simulink model "Project_4_Simulink"  (R2023b)
settings: Solver=ode45  StartTime=0.0  StopTime=3600  MaxStep=5.0  RelTol=1e-3
undefined symbols (not defined in the file or in its folder): batData, carData, motorData, track_radius
libraries: slpidlib x1
settings Model: NumberOfSteps=100  Creator=Matt Cain  LastModifiedBy=xavie

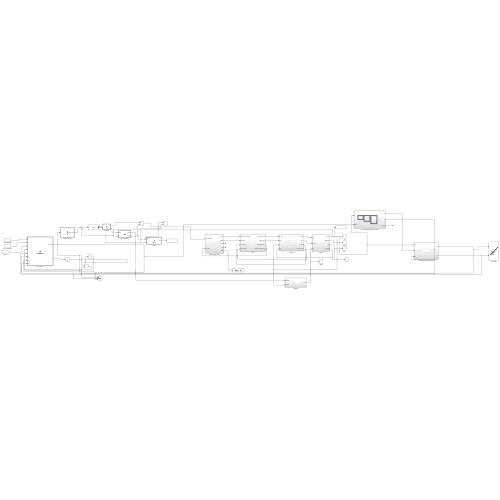
[thumbnail: Simulink's stored preview of the top-level diagram]
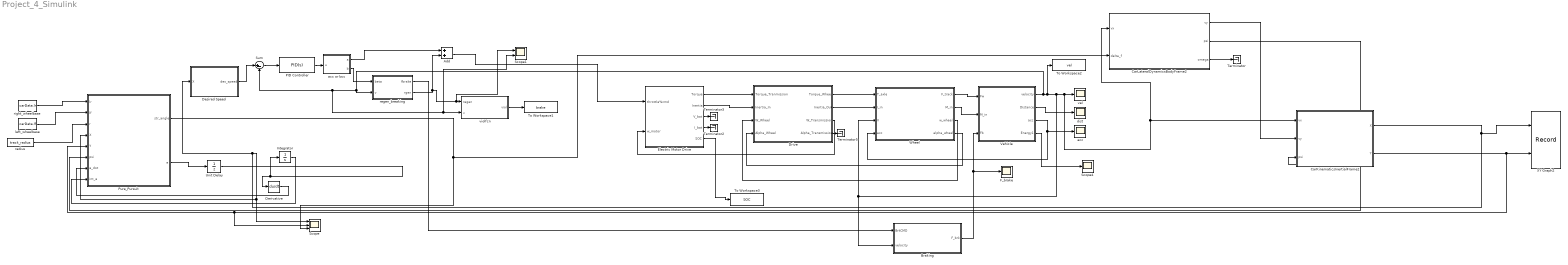
== system Project_4_Simulink ==
  Add : Sum
  Braking : Subsystem
  CarKinematicsInertialFrame2 : Subsystem
  CarLateralDynamicsBodyFrame2 : Subsystem
  Derivative : Derivative
  Desired Speed : MATLAB Function  TreatAsAtomicUnit=on
  Drive : Subsystem
  Electric Motor Drive : Subsystem
  F_brake : Scope
  Integrator : Integrator
  PID Controller : slpidlib/PID Controller  Controller=PID  Form=Parallel  TimeDomain=Continuous-time  UseExternalTs=off  SampleTime=-1  IntegratorMethod=Forward Euler  FilterMethod=Forward Euler  ControllerParametersSource=internal  P=0.1  I=0  UseKiTs=off  D=0  N=100  UseFilter=on  TunerSelectOption=Transfer Function Based (PID Tuner App)  InitialConditionSource=internal  InitialConditionForIntegrator=0  InitialConditionForFilter=0  DifferentiatorICPrevScaledInput=0  ExternalReset=none  TrackingMode=off  Kt=1  LimitOutput=on  SatLimitsSource=internal  UpperSaturationLimit=1  LowerSaturationLimit=-1  LinearizeAsGain=off  AntiWindupMode=none  Kb=1  LimitIntegrator=off  UpperIntegratorSaturationLimit=inf  LowerIntegratorSaturationLimit=-inf  POutMin=[]  POutMax=[]  IOutMin=[]  IOutMax=[]  DOutMin=[]  DOutMax=[]  NOutMin=[]  NOutMax=[]  SumOutMin=[]  SumOutMax=[]  SaturationOutMin=[]  SaturationOutMax=[]  PParamMin=[]  PParamMax=[]  IParamMin=[]  IParamMax=[]  DParamMin=[]  DParamMax=[]  NParamMin=[]  NParamMax=[]  KbParamMin=[]  KbParamMax=[]  KtParamMin=[]  KtParamMax=[]  KbOutMin=[]  KbOutMax=[]  KtOutMin=[]  KtOutMax=[]  IntegratorOutMin=[]  IntegratorOutMax=[]  FilterOutMin=[]  FilterOutMax=[]  SumI1OutMin=[]  SumI1OutMax=[]  SumI2OutMin=[]  SumI2OutMax=[]  SumI3OutMin=[]  SumI3OutMax=[]  SumI4OutMin=[]  SumI4OutMax=[]  SumDOutMin=[]  SumDOutMax=[]  DifferentiatorOutMin=[]  DifferentiatorOutMax=[]  FilterDiffOutCoefMin=[]  FilterDiffOutCoefMax=[]  ReciprocalOutMin=[]  ReciprocalOutMax=[]  SumDenOutMin=[]  SumDenOutMax=[]  SumNumOutMin=[]  SumNumOutMax=[]  DivideOutMin=[]  DivideOutMax=[]  UdiffTsProdOutMin=[]  UdiffTsProdOutMax=[]  NTsProdOutMin=[]  NTsProdOutMax=[]  UintegralTsProdOutMin=[]  UintegralTsProdOutMax=[]  UngainTsProdOutMin=[]  UngainTsProdOutMax=[]  ClampingZeroOutDataTypeStr=Inherit: Inherit via back propagation  ClampingZeroOutMin=[]  ClampingZeroOutMax=[]  FilterDenConstantOutDataTypeStr=Inherit: Inherit via back propagation  FilterDenConstantOutMin=[]  FilterDenConstantOutMax=[]  PCopyOutDataTypeStr=Inherit: Inherit via back propagation  PCopyOutMin=[]  PCopyOutMax=[]  NCopyOutDataTypeStr=Inherit: Inherit via back propagation  NCopyOutMin=[]  NCopyOutMax=[]  IntegratorContinuousStateAttributes=''  IntegratorStateMustResolveToSignalObject=off  IntegratorRTWStateStorageClass=Auto  FilterContinuousStateAttributes=''  FilterStateMustResolveToSignalObject=off  FilterRTWStateStorageClass=Auto  ParallelPVariant=InternalParameters  IdealPVariant=Disabled  IVariant=InternalParameters  DVariant=InternalParameters  IntegratorVariant=Continuous  SatVariant=Enabled  AWVariant=Passthrough  PCopyVariant=Disabled  TRVariant=Disabled  FdbkBlocksVariant=Forward  IdealPFdbkVariant=Disabled  SatFdbkVariant=Disabled  DerivativeFilterVariant=ContFilter  NVariant=InternalParameters  NCopyVariant=Disabled  FilterICVariant=InternalICsFilter  IntegratorICVariant=InternalICs  ExternalResetVariant=Disabled  TRSumVariant=Passthrough  SumFdbkVariant=Disabled  SumVariant=Sum_PID  TsampFilterVariant=InternalTs  TsampNgainVariant=Passthrough  TsampIntegralVariant=Disabled_SignalSpec  ExternalSaturationOutDataTypeStr=Inherit: Same as second input
  Pure_Pursuit : MATLAB Function  TreatAsAtomicUnit=on
  Scope : Scope  NumInputPorts=3
  Scope1 : Scope  NumInputPorts=2
  Scope4 : Scope
  Sum : Sum  Inputs=|+-
  Terminator{,2..3,5} (4 alike) : Terminator
  To Workspace1 : ToWorkspace  VariableName=brake  SaveFormat=Timeseries  SampleTime=-1
  To Workspace2 : ToWorkspace  VariableName=vel  SaveFormat=Timeseries  SampleTime=-1
  To Workspace3 : ToWorkspace  VariableName=SOC  SaveFormat=Timeseries  SampleTime=-1
  Unit Delay : UnitDelay  SampleTime=-1  HasFrameUpgradeWarning=on
  Vehicle : Subsystem
  "Wheel " : Subsystem
  XY Graph2 : Record  FileSettingsInternal="{\"entries\":[{\"content\":{\"excelSettings\":{\"content\":{},\"type\":\"Streamout.ExcelSettings\"}},\"type\":\"Streamout.FileSettingStorage\",\"uuid\":\"\"}],\"packageUris\":[\"http:\\/\\/schema.mathworks.com\\/mf0\\/streamout_blocks\\/R2020a\"],\"version\":\"1.0\"}"  Layout=[1 1]  SignalsInternal="{\"entries\":[{\"content\":{\"signals\":[{\"content\":{\"blockPath\":[],\"dimensions\":[1],\"domain\":\"\",\"lineColor\":\"#edb120\",\"port\":1,\"sid\":[\"\"],\"signalID\":23658,\"signalName\":\"CarKinematicsInertialFrame2:1\"},\"type\":\"RecordBlkView.Signal\",\"uuid\":\"\"},{\"content\":{\"blockPath\":[],\"dimensions\":[1],\"domain\":\"\",\"lineColor\":\"#7e2f8e\",\"port\":2,\"sid\":[\"\"],\"signalID\":23662,\"signalName\":\"CarKinematicsInertialFrame2:2\"},\"type\":\"RecordBlkView.Signal\",\"uuid\":\"\"}]},\"type\":\"RecordBlkView.InputSignals\",\"uuid\":\"\"}],\"packageUris\":[\"http:\\/\\/schema.mathworks.com\\/mf0\\/streamout_blocks\\/R2020a\"],\"version\":\"1.0\"}"  VisualizationBindings="{\"xyplotplugin\":{\"info\":[{\"series\":[{\"bindingParametersList\":[{\"parameter\":\"X-Axis\",\"signalID\":23062,\"signalName\":\"CarKinematicsInertialFrame2:1\"},{\"parameter\":\"Y-Axis\",\"signalID\":23066,\"signalName\":\"CarKinematicsInertialFrame2:2\"}],\"seriesID\":49385}],\"subplotID\":1}]}}"  CompatibilityTag=XY  st=-1
  acc : Scope
  acc or bcc : MATLAB Function  TreatAsAtomicUnit=on
  dist : Scope
  left_wheelbase : Constant  Value=carData.lf
  radius : Constant  Value=track_radius
  regen_breaking : MATLAB Function  TreatAsAtomicUnit=on
  right_wheelbase : Constant  Value=carData.lr
  vel : Scope
  violfcn : MATLAB Function  TreatAsAtomicUnit=on
  wires:
  acc or bcc/2(b) -> regen_breaking/1(beta)
  CarKinematicsInertialFrame2/1(X) -> Desired Speed/1(X), Scope/1, Pure_Pursuit/4(X), XY Graph2/1
  regen_breaking/2(rgen) -> Add/2, Scope1/1, violfcn/1(regen)
  Pure_Pursuit/1(str_angle) -> CarLateralDynamicsBodyFrame2/2(delta_f), Scope/3
  Sum/1 -> PID Controller/1
  violfcn/1(viol) -> To Workspace1/1
  Integrator/1 -> Pure_Pursuit/8(int_e)
  right_wheelbase/1 -> Pure_Pursuit/1(lr)
  CarLateralDynamicsBodyFrame2/2(psi) -> Pure_Pursuit/6(psi), CarKinematicsInertialFrame2/3(psi)
  CarKinematicsInertialFrame2/2(Y) -> XY Graph2/2, Pure_Pursuit/5(Y), Scope/2
  Pure_Pursuit/2(e) -> Unit Delay/1
  left_wheelbase/1 -> Pure_Pursuit/2(lf)
  Unit Delay/1 -> Derivative/1, Integrator/1
  acc or bcc/1(a) -> Add/1
  Derivative/1 -> Pure_Pursuit/7(e_dot)
  radius/1 -> Pure_Pursuit/3(r)
  Vehicle/1("velocity ") -> Sum/2, Scope1/2, violfcn/2(v), regen_breaking/2(v), To Workspace2/1, CarLateralDynamicsBodyFrame2/1(vx), CarKinematicsInertialFrame2/1(vx), vel/1, Braking/2("velocity "), "Wheel "/3(V)
  PID Controller/1 -> acc or bcc/1(u)
  Desired Speed/1(des_speed) -> Sum/1
  "Wheel "/3(w_wheel) -> Drive/3(W_Wheel)
  regen_breaking/1(fbrake) -> Braking/1("BrkCMD ")
  "Wheel "/4(alpha_wheel) -> Drive/4(Alpha_Wheel)
  Drive/4(Alpha_Transmission) -> Terminator5/1
  "Wheel "/2(M_in) -> Vehicle/2("M_in ")
  Electric Motor Drive/5(SOC) -> To Workspace3/1
  Vehicle/2("Distance ") -> dist/1
  Electric Motor Drive/2(Inertia) -> Drive/2(Inertia_In)
  Electric Motor Drive/4(I_bat) -> Terminator2/1
  Electric Motor Drive/1(Torque) -> Drive/1(Torque_Tranmission)
  Vehicle/3(acc) -> acc/1, "Wheel "/4(acc)
  "Wheel "/1(F_track) -> Vehicle/1("Fw ")
  Drive/3(W_Transmission) -> Electric Motor Drive/2(w_motor)
  Electric Motor Drive/3(V_bat) -> Terminator3/1
  Braking/1("F_brk ") -> Vehicle/3("Fb "), F_brake/1
  Drive/2(Inertia_Out) -> "Wheel "/2(I_in)
  Drive/1(Torque_Wheel) -> "Wheel "/1(T_axle)
  CarLateralDynamicsBodyFrame2/1(vy) -> CarKinematicsInertialFrame2/2(vy)
  Add/1 -> Electric Motor Drive/1(throttle%cmd)
  CarLateralDynamicsBodyFrame2/3(omega) -> Terminator/1
  Vehicle/4(Energy1) -> Scope4/1

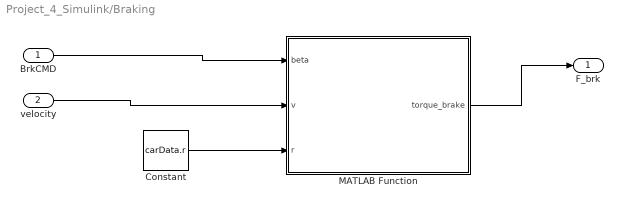
== system Project_4_Simulink/Braking ==
  "BrkCMD " : Inport
  "velocity " : Inport  Port=2
  Constant : Constant  Value=carData.r
  MATLAB Function : MATLAB Function  TreatAsAtomicUnit=on
  "F_brk " : Outport  VectorParamsAs1DForOutWhenUnconnected=off
  wires:
  "BrkCMD "/1 -> MATLAB Function/1(beta)
  MATLAB Function/1(torque_brake) -> "F_brk "/1
  "velocity "/1 -> MATLAB Function/2(v)
  Constant/1 -> MATLAB Function/3(r)

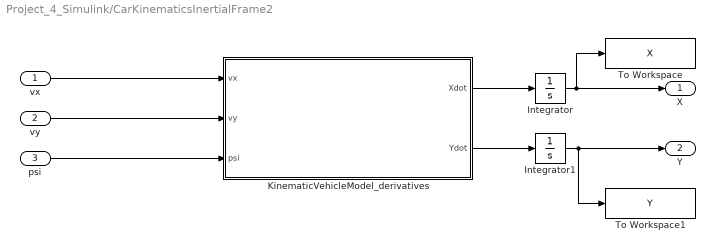
== system Project_4_Simulink/CarKinematicsInertialFrame2 ==
  vx : Inport
  vy : Inport  Port=2
  psi : Inport  Port=3
  Integrator : Integrator  InitialCondition=carData.init.X0
  Integrator1 : Integrator  InitialCondition=carData.init.Y0
  KinematicVehicleModel_derivatives : MATLAB Function  TreatAsAtomicUnit=on  mask{obj=carData}
      mask prompts: obj "obj structure"
  To Workspace : ToWorkspace  VariableName=X  SaveFormat=Structure With Time  SampleTime=-1
  To Workspace1 : ToWorkspace  VariableName=Y  SaveFormat=Structure With Time  SampleTime=-1
  X : Outport
  Y : Outport  Port=2
  wires:
  KinematicVehicleModel_derivatives/1(Xdot) -> Integrator/1
  KinematicVehicleModel_derivatives/2(Ydot) -> Integrator1/1
  Integrator/1 -> To Workspace/1, X/1
  Integrator1/1 -> To Workspace1/1, Y/1
  vx/1 -> KinematicVehicleModel_derivatives/1(vx)
  vy/1 -> KinematicVehicleModel_derivatives/2(vy)
  psi/1 -> KinematicVehicleModel_derivatives/3(psi)

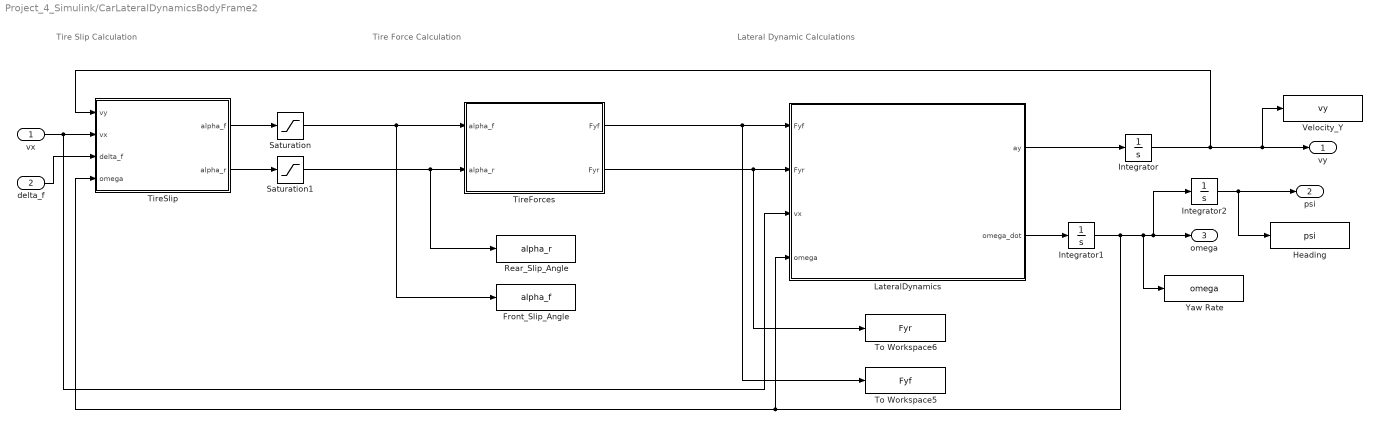
== system Project_4_Simulink/CarLateralDynamicsBodyFrame2 ==
  note: Tire Slip Calculation
  note: Tire Force Calculation
  note: Lateral Dynamic Calculations
  vx : Inport
  delta_f : Inport  Port=2
  Front_Slip_Angle : ToWorkspace  VariableName=alpha_f  SaveFormat=Timeseries  SampleTime=-1
  Heading : ToWorkspace  VariableName=psi  SaveFormat=Timeseries  SampleTime=-1
  Integrator : Integrator  InitialCondition=carData.init.vy0
  Integrator1 : Integrator  InitialCondition=carData.init.omega0
  Integrator2 : Integrator  InitialCondition=carData.init.psi0
  LateralDynamics : MATLAB Function  TreatAsAtomicUnit=on  mask{obj=carData}
      mask prompts: obj "obj structure"
  Rear_Slip_Angle : ToWorkspace  VariableName=alpha_r  SaveFormat=Timeseries  SampleTime=-1
  Saturation : Saturate  UpperLimit=carData.maxAlpha  LowerLimit=-carData.maxAlpha
  Saturation1 : Saturate  UpperLimit=carData.maxAlpha  LowerLimit=-carData.maxAlpha
  TireForces : MATLAB Function  TreatAsAtomicUnit=on  mask{obj=carData}
      mask prompts: obj "obj structure"
  TireSlip : MATLAB Function  TreatAsAtomicUnit=on  mask{obj=carData}
      mask prompts: obj "obj structure"
  To Workspace5 : ToWorkspace  VariableName=Fyf  SaveFormat=Timeseries  SampleTime=-1
  To Workspace6 : ToWorkspace  VariableName=Fyr  SaveFormat=Timeseries  SampleTime=-1
  Velocity_Y : ToWorkspace  VariableName=vy  SaveFormat=Timeseries  SampleTime=-1
  Yaw Rate : ToWorkspace  VariableName=omega  SaveFormat=Timeseries  SampleTime=-1
  vy : Outport
  psi : Outport  Port=2
  omega : Outport  Port=3
  wires:
  LateralDynamics/1(ay) -> Integrator/1
  Integrator/1 -> vy/1, Velocity_Y/1, TireSlip/1(vy)
  LateralDynamics/2(omega_dot) -> Integrator1/1
  Integrator1/1 -> Integrator2/1, omega/1, Yaw Rate/1, LateralDynamics/4(omega), TireSlip/4(omega)
  TireSlip/1(alpha_f) -> Saturation/1
  TireSlip/2(alpha_r) -> Saturation1/1
  TireForces/1(Fyf) -> LateralDynamics/1(Fyf), To Workspace5/1
  TireForces/2(Fyr) -> LateralDynamics/2(Fyr), To Workspace6/1
  Saturation/1 -> TireForces/1(alpha_f), Front_Slip_Angle/1
  Saturation1/1 -> TireForces/2(alpha_r), Rear_Slip_Angle/1
  vx/1 -> TireSlip/2(vx), LateralDynamics/3(vx)
  delta_f/1 -> TireSlip/3(delta_f)
  Integrator2/1 -> Heading/1, psi/1

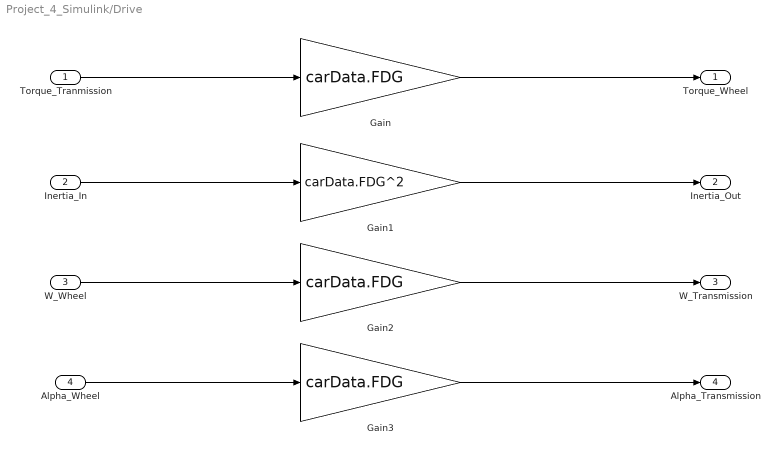
== system Project_4_Simulink/Drive ==
  Torque_Tranmission : Inport
  Inertia_In : Inport  Port=2
  W_Wheel : Inport  Port=3
  Alpha_Wheel : Inport  Port=4
  Gain : Gain  Gain=carData.FDG
  Gain1 : Gain  Gain=carData.FDG^2
  Gain2 : Gain  Gain=carData.FDG
  Gain3 : Gain  Gain=carData.FDG
  Torque_Wheel : Outport
  Inertia_Out : Outport  Port=2
  W_Transmission : Outport  Port=3
  Alpha_Transmission : Outport  Port=4
  wires:
  Torque_Tranmission/1 -> Gain/1
  Inertia_In/1 -> Gain1/1
  W_Wheel/1 -> Gain2/1
  Alpha_Wheel/1 -> Gain3/1
  Gain/1 -> Torque_Wheel/1
  Gain1/1 -> Inertia_Out/1
  Gain2/1 -> W_Transmission/1
  Gain3/1 -> Alpha_Transmission/1

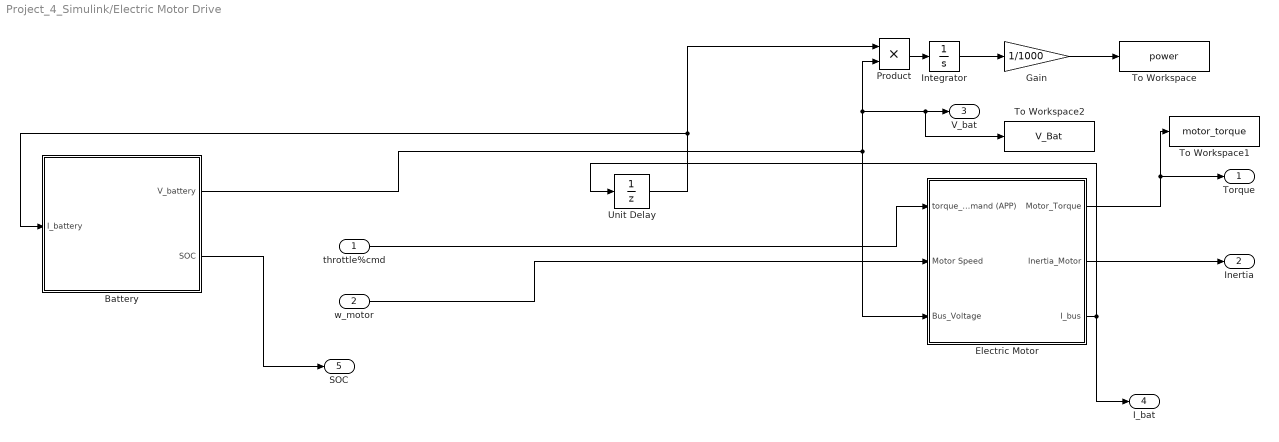
== system Project_4_Simulink/Electric Motor Drive ==
  throttle%cmd : Inport
  w_motor : Inport  Port=2
  Battery : Subsystem
  Electric Motor : Subsystem
  Gain : Gain  Gain=1/1000
  Integrator : Integrator
  Product : Product
  To Workspace : ToWorkspace  VariableName=power  SaveFormat=Timeseries  SampleTime=-1
  To Workspace1 : ToWorkspace  VariableName=motor_torque  SaveFormat=Timeseries  SampleTime=-1
  To Workspace2 : ToWorkspace  VariableName=V_Bat  SaveFormat=Timeseries  SampleTime=-1
  Unit Delay : UnitDelay  SampleTime=-1  HasFrameUpgradeWarning=on
  Torque : Outport
  Inertia : Outport  Port=2
  V_bat : Outport  Port=3
  I_bat : Outport  Port=4
  SOC : Outport  Port=5
  wires:
  throttle%cmd/1 -> Electric Motor/1(torque_Command (APP))
  w_motor/1 -> Electric Motor/2(Motor Speed)
  Electric Motor/3(I_bus) -> Unit Delay/1, I_bat/1
  Battery/1(V_battery) -> To Workspace2/1, V_bat/1, Product/2, Electric Motor/3(Bus_Voltage)
  Battery/2(SOC) -> SOC/1
  Electric Motor/2(Inertia_Motor) -> Inertia/1
  Electric Motor/1(Motor_Torque) -> To Workspace1/1, Torque/1
  Unit Delay/1 -> Battery/1(I_battery), Product/1
  Product/1 -> Integrator/1
  Integrator/1 -> Gain/1
  Gain/1 -> To Workspace/1

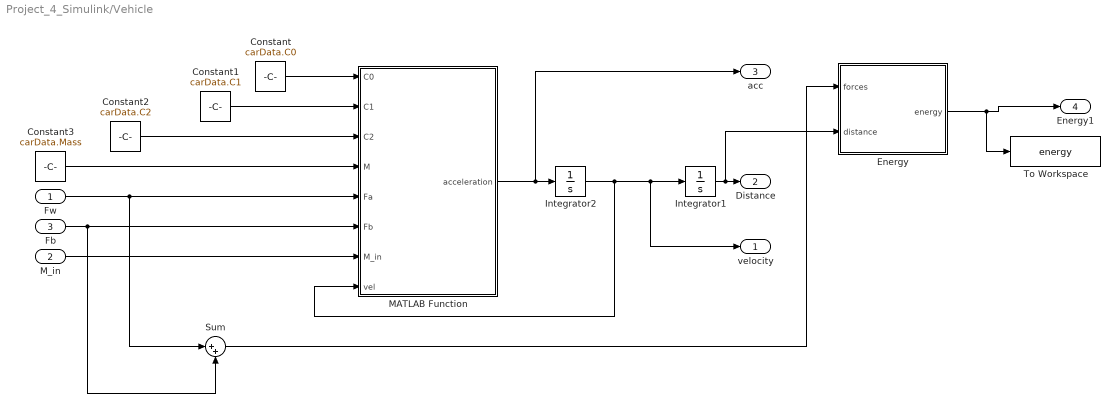
== system Project_4_Simulink/Vehicle ==
  "Fw " : Inport
  "M_in " : Inport  Port=2
  "Fb " : Inport  Port=3
  Constant : Constant  Value=carData.C0
  Constant1 : Constant  Value=carData.C1
  Constant2 : Constant  Value=carData.C2
  Constant3 : Constant  Value=carData.Mass
  Energy : MATLAB Function  TreatAsAtomicUnit=on
  Integrator1 : Integrator
  Integrator2 : Integrator  LimitOutput=on  LowerSaturationLimit=0
  MATLAB Function : MATLAB Function  TreatAsAtomicUnit=on
  Sum : Sum  Inputs=|++
  To Workspace : ToWorkspace  VariableName=energy  SaveFormat=Timeseries  SampleTime=-1
  "velocity " : Outport  VectorParamsAs1DForOutWhenUnconnected=off
  "Distance " : Outport  Port=2  VectorParamsAs1DForOutWhenUnconnected=off
  acc : Outport  Port=3
  Energy1 : Outport  Port=4
  wires:
  Constant1/1 -> MATLAB Function/2(C1)
  Constant/1 -> MATLAB Function/1(C0)
  Constant2/1 -> MATLAB Function/3(C2)
  Constant3/1 -> MATLAB Function/4(M)
  "Fw "/1 -> Sum/1, MATLAB Function/5(Fa)
  "Fb "/1 -> Sum/2, MATLAB Function/6(Fb)
  Integrator1/1 -> Energy/2(distance), "Distance "/1
  "M_in "/1 -> MATLAB Function/7(M_in)
  MATLAB Function/1(acceleration) -> acc/1, Integrator2/1
  Integrator2/1 -> MATLAB Function/8(vel), "velocity "/1, Integrator1/1
  Sum/1 -> Energy/1(forces)
  Energy/1(energy) -> To Workspace/1, Energy1/1

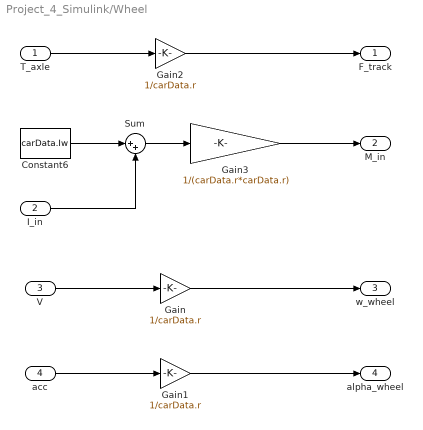
== system Project_4_Simulink/Wheel  ==
  T_axle : Inport
  I_in : Inport  Port=2
  V : Inport  Port=3
  acc : Inport  Port=4
  Constant6 : Constant  Value=carData.Iw
  Gain : Gain  Gain=1/carData.r
  Gain1 : Gain  Gain=1/carData.r
  Gain2 : Gain  Gain=1/carData.r
  Gain3 : Gain  Gain=1/(carData.r*carData.r)
  Sum : Sum  Inputs=|++
  F_track : Outport
  M_in : Outport  Port=2
  w_wheel : Outport  Port=3
  alpha_wheel : Outport  Port=4
  wires:
  Gain/1 -> w_wheel/1
  V/1 -> Gain/1
  acc/1 -> Gain1/1
  Gain1/1 -> alpha_wheel/1
  T_axle/1 -> Gain2/1
  Gain2/1 -> F_track/1
  Gain3/1 -> M_in/1
  Constant6/1 -> Sum/1
  I_in/1 -> Sum/2
  Sum/1 -> Gain3/1

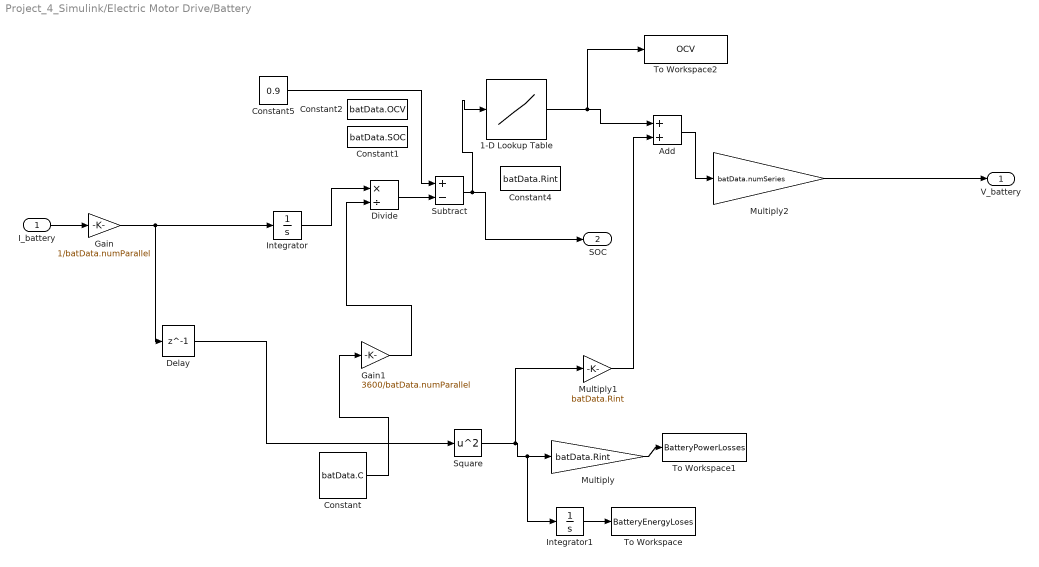
== system Project_4_Simulink/Electric Motor Drive/Battery ==
  I_battery : Inport
  1-D Lookup Table : Lookup_n-D  NumberOfTableDimensions=1  BreakpointsForDimension1=batData.SOC  Table=batData.OCV  InternalRulePriority=Speed  RndMeth=Simplest
  Add : Sum
  Constant : Constant  Value=batData.C
  Constant1 : Constant  Value=batData.SOC
  Constant2 : Constant  Value=batData.OCV
  Constant4 : Constant  Value=batData.Rint
  Constant5 : Constant  Value=0.9
  Delay : Delay  DelayLength=1
  Divide : Product  Inputs=*/
  Gain : Gain  Gain=1/batData.numParallel
  Gain1 : Gain  Gain=3600/batData.numParallel
  Integrator : Integrator
  Integrator1 : Integrator
  Multiply : Gain  Gain=batData.Rint
  Multiply1 : Gain  Gain=batData.Rint
  Multiply2 : Gain  Gain=batData.numSeries
  Square : Math  Operator=square
  Subtract : Sum  Inputs=+-
  To Workspace : ToWorkspace  VariableName=BatteryEnergyLoses  SaveFormat=Timeseries  SampleTime=-1
  To Workspace1 : ToWorkspace  VariableName=BatteryPowerLosses  SaveFormat=Timeseries  SampleTime=-1
  To Workspace2 : ToWorkspace  VariableName=OCV  SaveFormat=Timeseries  SampleTime=-1
  V_battery : Outport
  SOC : Outport  Port=2
  wires:
  I_battery/1 -> Gain/1
  Gain/1 -> Delay/1, Integrator/1
  Integrator/1 -> Divide/1
  Constant/1 -> Gain1/1
  Gain1/1 -> Divide/2
  Divide/1 -> Subtract/2
  Constant5/1 -> Subtract/1
  Subtract/1 -> 1-D Lookup Table/1, SOC/1
  Delay/1 -> Square/1
  Square/1 -> Multiply1/1, Integrator1/1, Multiply/1
  1-D Lookup Table/1 -> To Workspace2/1, Add/1
  Multiply1/1 -> Add/2
  Add/1 -> Multiply2/1
  Integrator1/1 -> To Workspace/1
  Multiply/1 -> To Workspace1/1
  Multiply2/1 -> V_battery/1

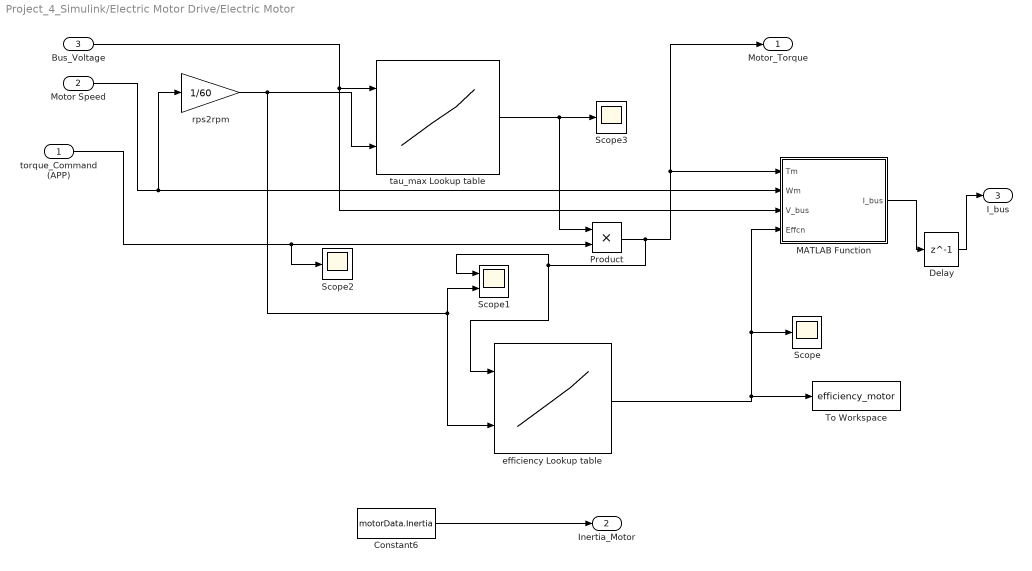
== system Project_4_Simulink/Electric Motor Drive/Electric Motor ==
  torque_Command (APP) : Inport
  Motor Speed : Inport  Port=2
  Bus_Voltage : Inport  Port=3
  Constant6 : Constant  Value=motorData.Inertia
  Delay : Delay  DelayLength=1
  MATLAB Function : MATLAB Function  TreatAsAtomicUnit=on
  Product : Product
  Scope : Scope
  Scope1 : Scope  NumInputPorts=2
  Scope2 : Scope
  Scope3 : Scope
  To Workspace : ToWorkspace  VariableName=efficiency_motor  SaveFormat=Timeseries  SampleTime=-1
  efficiency Lookup table : Lookup_n-D  BreakpointsForDimension1=motorData.eta_torque  BreakpointsForDimension2=motorData.eta_speed  BeginIndexSearchUsingPreviousIndexResult=on  Table=motorData.eta_val  InternalRulePriority=Speed  RndMeth=Simplest
      settings: InputPortMap=u0,u1
  rps2rpm : Gain  Gain=1/60
  tau_max Lookup table : Lookup_n-D  BreakpointsForDimension1=motorData.vbus  BreakpointsForDimension2=motorData.rpm  Table=motorData.maxtorque  InternalRulePriority=Speed  RndMeth=Simplest
      settings: InputPortMap=u0,u1
  Motor_Torque : Outport
  Inertia_Motor : Outport  Port=2
  I_bus : Outport  Port=3
  wires:
  Bus_Voltage/1 -> tau_max Lookup table/1, MATLAB Function/3(V_bus)
  torque_Command (APP)/1 -> Scope2/1, Product/2
  tau_max Lookup table/1 -> Product/1, Scope3/1
  Product/1 -> efficiency Lookup table/1, Scope1/1, MATLAB Function/1(Tm), Motor_Torque/1
  efficiency Lookup table/1 -> MATLAB Function/4(Effcn), Scope/1, To Workspace/1
  MATLAB Function/1(I_bus) -> Delay/1
  Constant6/1 -> Inertia_Motor/1
  Motor Speed/1 -> MATLAB Function/2(Wm), rps2rpm/1
  rps2rpm/1 -> Scope1/2, efficiency Lookup table/2, tau_max Lookup table/2
  Delay/1 -> I_bus/1

== matlab function Project_4_Simulink/CarLateralDynamicsBodyFrame2/LateralDynamics ==
  data: Fyf input; Fyr input size=1; vx input; omega input; ay output; obj parameter; omega_dot output
function [ay, omega_dot] = fcn(Fyf, Fyr, vx, omega, obj)

Fy = Fyf + Fyr;
ay = Fy / obj.Mass - omega * vx;
        
M  = Fyf * obj.lf - Fyr * obj.lr;        
omega_dot = M / obj.Inertia;        

end

== matlab function Project_4_Simulink/CarLateralDynamicsBodyFrame2/TireForces ==
  data: alpha_f input; alpha_r input; Fyf output; obj parameter; Fyr output
function [Fyf, Fyr] = fcn(alpha_f, alpha_r, obj)

Fyf = min(obj.Fyfmax,obj.Calpha_f * alpha_f);
Fyr = min(obj.Fyrmax, obj.Calpha_r * alpha_r);
end

== matlab function Project_4_Simulink/CarLateralDynamicsBodyFrame2/TireSlip ==
  data: vy input size=1; vx input; delta_f input size=1; omega input; alpha_f output; obj parameter; alpha_r output
function [alpha_f, alpha_r] = fcn(vy,  vx, delta_f, omega, obj)


if abs(vx)> obj.vx_threshold1
      alpha_f = delta_f - (vy + omega * obj.lf) / vx;
      alpha_r = - (vy - omega * obj.lr) / vx;
else
      alpha_f = 0;
      alpha_r = 0;
end



end

== matlab function Project_4_Simulink/CarKinematicsInertialFrame2/KinematicVehicleModel_derivatives ==
  data: vx input; vy input; psi input size=1; Xdot output; Ydot output
function [Xdot, Ydot] = fcn(vx, vy, psi)
    temp = TF(psi) * [vx;vy]; 
    Xdot = temp(1);
    Ydot = temp(2);
  
end

function y = TF(psi)
    y = [cos(psi), -sin(psi); sin(psi), cos(psi)];
end

== matlab function Project_4_Simulink/acc or bcc ==
  data: u input; a output; b output
% Checks if there is a difference between actual speed and desired speed

% u is calculated using the sum function in the simulink model

function [a,b] = fcn(u)

if u>0 % If the difference is greater than zero, then we need to speed up since actual speed is less than desired speed
    acc=u; % We send how much we need to speed up to the throttle command
    brk=0; % Do nothing for the break command
elseif u<0 % If the difference is less than zero, then we need to slow down since the actual speed is less than the desired speed
    acc=0; % Do nothing for throttle command
    brk=-u; % We send how much we need to break to the break command
else % If the desired and actual speed is the same
    acc=0; % Do nothing for throttle command
    brk=0; % Do nothing for the break command
end
a= acc; % storing how much acceleration required to a
b= brk; % storing how much break acceleration required to b

== matlab function Project_4_Simulink/Pure_Pursuit ==
  data: lr input; lf input; r input; X input; str_angle output; Y input; psi input; e_dot input; int_e input; e output
function [str_angle, e] = SimplestDriver(lr, lf, r, X, Y, psi, e_dot, int_e)
lookout = 10;
kp = .0017;
kd = 0;
ki = 0;
if X >= 900
    theta = atan(200-Y/X-900);
    psi_desired = psi+theta;
    e = psi - psi_desired;
    PID = kp*e + kd*e_dot + ki*int_e;
    str_angle = PID + (lr+lf)/r;
elseif X < 0
    theta = atan(200-Y/X - 900);
    psi_desired = psi+theta;
    e = psi - psi_desired;
    PID = kp*e + kd*e_dot + ki*int_e;
    str_angle = PID + (lr+lf)/r;
else
    str_angle = 0;
    psi_desired = 0;
    e = psi-psi_desired;
    kp = 0.00050;
    kd = 0.0007/1000000;
    ki = 0.00000000011/100000000;
    if Y < 200
        lookout= 45;
        vertical = -Y;
        psi_desired = atan(vertical/lookout);
        e = psi_desired;
        PID = kp*e + kd*e_dot + ki*int_e;
        str_angle = PID;
    end
    if Y > 200
        lookout= -45;
        vertical = 400-Y;
        psi_desired = atan(vertical/lookout);
        e = psi_desired;
        PID = kp*e + kd*e_dot + ki*int_e;
        str_angle = PID;
    end
end

== matlab function Project_4_Simulink/Desired Speed ==
  data: X input; des_speed output
function des_speed = fcn(X)
if X > 0  && X <15 || X < 900 && X > 885
    des_speed = 70;
elseif X <= 885 && X >= 15
    des_speed = 80;
else
    des_speed = 10.5;
end

== matlab function Project_4_Simulink/violfcn ==
  data: regen input; viol output; v input

function viol = violfcn(regen, v)
    speed = v ;%* (3600/1600);
    if speed < 5
        regen_vio = 0;
        if abs(regen -regen_vio ) < 1E-6
            viol = 0;
        else
            viol = 1;
        end

    elseif speed == 25
        regen_vio = 0.95;
        if abs(regen - regen_vio ) < 1E-6
            viol = 0;
        else
            viol = 1;
        end

    elseif speed > 25
        regen_vio = 0.95;
        if abs(regen -regen_vio ) < 1E-6
            viol = 0;
        else
            viol = 1;
        end
    else
        regen_vio = ((0.95/20)*speed) - 0.2375;
        if abs(regen -regen_vio ) < 1E-6
            viol = 0;
        else
            viol = 1;
        end
    end

== matlab function Project_4_Simulink/regen_breaking ==
  data: fbrake output; beta input; v input; rgen output
% function [fbrake, rgen] = fcn(beta, v)
function [fbrake, rgen]= fcn(beta, v)
%speed = v * (3600/1600);
%v = speed;
if v <= 5
    rgen = 0;
    fbrake = beta;
elseif v > 5
    rgen = .0475 * ((v-5)*beta);
    fbrake = ( 1-0.0475)*((v-5)*beta);
else
    rgen = 0.05*beta;
    fbrake = 0.95*beta;
end

== matlab function Project_4_Simulink/Braking/MATLAB Function ==
  data: beta input; torque_brake output; v input; r input

function torque_brake = torque_brake(beta,v,r)
if beta == 0
    torque_brake = 0;
else
    torque_brake = beta * 10000 * (v / abs(v)+0.001) /r;
end

== matlab function Project_4_Simulink/Vehicle/Energy ==
  data: forces input; energy output; distance input
function energy = fcn(forces, distance)

energy = dot(forces, distance);

== matlab function Project_4_Simulink/Electric Motor Drive/Electric Motor/MATLAB Function ==
  data: Tm input; I_bus output; Wm input; V_bus input; Effcn input
function I_bus = fcn(Tm,Wm,V_bus,Effcn)

Pm = Tm * Wm;
sgn_Pm = Pm/(abs(Pm)+0.001);
Pe = Pm * Effcn^(complex(sgn_Pm)); 
I_bus = real(Pe)/V_bus; % Calculating I_bus

== matlab function Project_4_Simulink/Vehicle/MATLAB Function ==
  data: C0 input; acceleration output; C1 input; C2 input; M input; Fa input; Fb input; M_in input; vel input
function acceleration   = vehicle(C0,C1,C2,M,Fa,Fb,M_in, vel)

acceleration = (((Fa-Fb))-(C0+ C1*vel + C2*(vel)^2))/(M+M_in);
